simulink library "Eclipse"  (R2014b)
settings: Solver=ode45  StartTime=0.0  StopTime=10.0  RelTol=1e-3
undefined symbols (not defined in the file): ConfParam
settings Model: Creator=Hp  LastModifiedBy=Hp

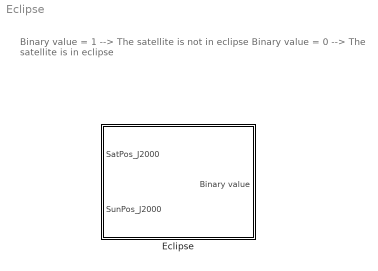
== system Eclipse ==
  note: Binary value = 1 --> The satellite is not in eclipse
      |
      | Binary value = 0 --> The satellite is in eclipse
  Eclipse : Subsystem

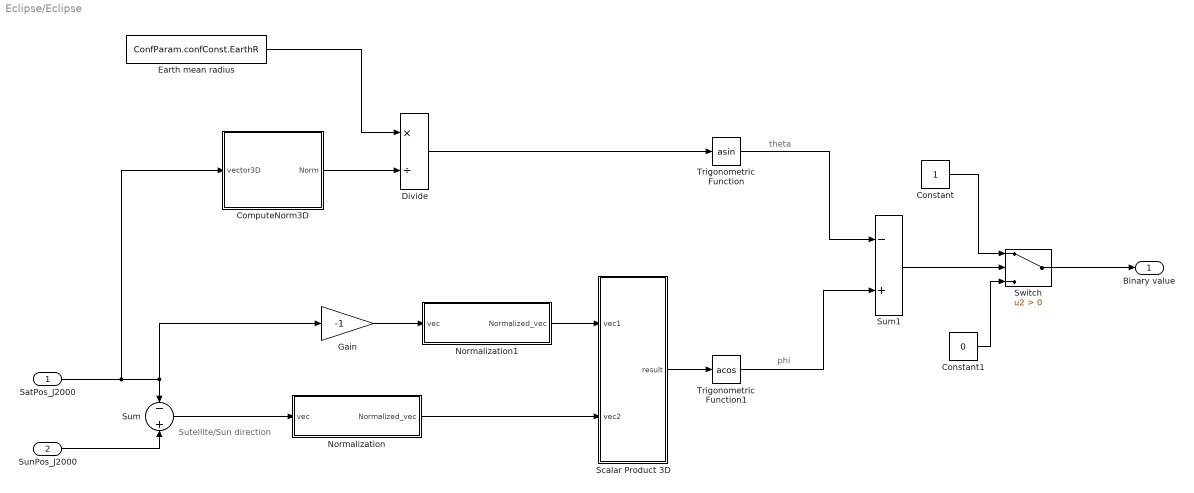
== system Eclipse/Eclipse ==
  note: phi
  note: theta
  note: Sutellite/Sun direction
  SatPos_J2000 : Inport
  SunPos_J2000 : Inport  Port=2
  ComputeNorm3D : Subsystem
  Constant : Constant
  Constant1 : Constant  Value=0
  Divide : Product  Inputs=*/
  Earth mean radius : Constant  Value=ConfParam.confConst.EarthR
  Gain : Gain  Gain=-1
  Normalization : Subsystem
  Normalization1 : Subsystem
  Scalar Product 3D : Subsystem
  Sum : Sum  Inputs=-|+
  Sum1 : Sum  Inputs=-+
  Switch : Switch  Criteria=u2 > Threshold
  Trigonometric Function : Trigonometry  Operator=asin
  Trigonometric Function1 : Trigonometry  Operator=acos
  Binary value : Outport
  wires:
  SatPos_J2000/1 -> ComputeNorm3D/1(vector3D), Sum/1, Gain/1
  SunPos_J2000/1 -> Sum/2
  Earth mean radius/1 -> Divide/1
  ComputeNorm3D/1(Norm) -> Divide/2
  Divide/1 -> Trigonometric Function/1
  Scalar Product 3D/1(result) -> Trigonometric Function1/1
  Sum/1 -> Normalization/1(vec)
  Normalization1/1(Normalized_vec) -> Scalar Product 3D/1(vec1)
  Normalization/1(Normalized_vec) -> Scalar Product 3D/2(vec2)
  Gain/1 -> Normalization1/1(vec)
  Switch/1 -> Binary value/1
  Trigonometric Function1/1 -> Sum1/2
  Constant/1 -> Switch/1
  Constant1/1 -> Switch/3
  Sum1/1 -> Switch/2
  Trigonometric Function/1 -> Sum1/1

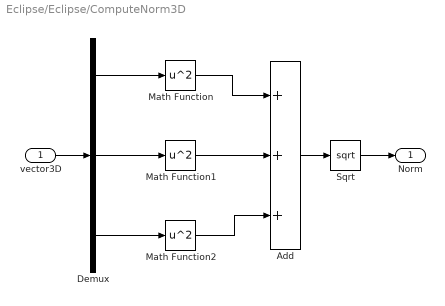
== system Eclipse/Eclipse/ComputeNorm3D ==
  vector3D : Inport
  Add : Sum  Inputs=+++
  Demux : Demux  Outputs=3
  Math Function : Math  Operator=square  SaturateOnIntegerOverflow=on
  Math Function1 : Math  Operator=square  SaturateOnIntegerOverflow=on
  Math Function2 : Math  Operator=square  SaturateOnIntegerOverflow=on
  Sqrt : Sqrt  SaturateOnIntegerOverflow=on
  Norm : Outport
  wires:
  vector3D/1 -> Demux/1
  Sqrt/1 -> Norm/1
  Add/1 -> Sqrt/1
  Math Function1/1 -> Add/2
  Math Function2/1 -> Add/3
  Demux/1 -> Math Function/1
  Math Function/1 -> Add/1
  Demux/3 -> Math Function2/1
  Demux/2 -> Math Function1/1

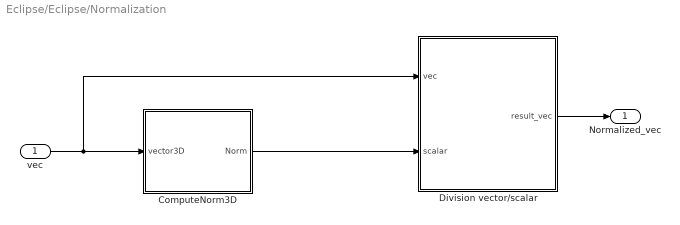
== system Eclipse/Eclipse/Normalization ==
  vec : Inport
  ComputeNorm3D : Subsystem
  Division vector/scalar : Subsystem
  Normalized_vec : Outport
  wires:
  vec/1 -> Division vector/scalar/1(vec), ComputeNorm3D/1(vector3D)
  Division vector/scalar/1(result_vec) -> Normalized_vec/1
  ComputeNorm3D/1(Norm) -> Division vector/scalar/2(scalar)

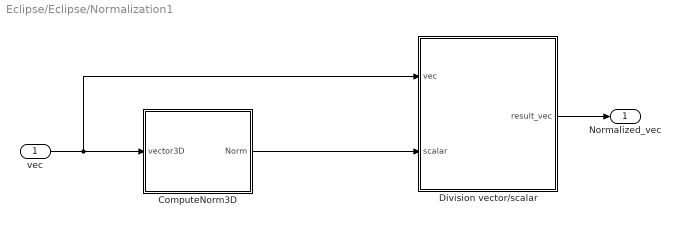
== system Eclipse/Eclipse/Normalization1 ==
  vec : Inport
  ComputeNorm3D : Subsystem
  Division vector/scalar : Subsystem
  Normalized_vec : Outport
  wires:
  vec/1 -> Division vector/scalar/1(vec), ComputeNorm3D/1(vector3D)
  Division vector/scalar/1(result_vec) -> Normalized_vec/1
  ComputeNorm3D/1(Norm) -> Division vector/scalar/2(scalar)

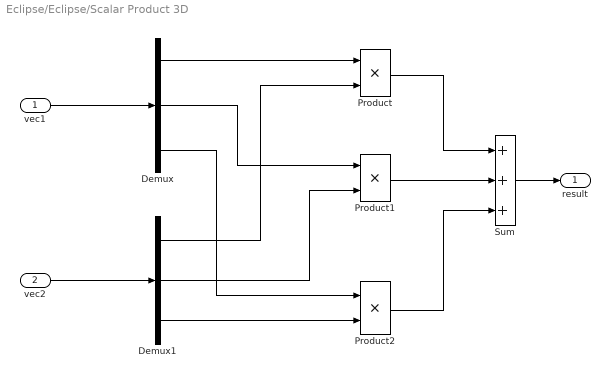
== system Eclipse/Eclipse/Scalar Product 3D ==
  vec1 : Inport
  vec2 : Inport  Port=2
  Demux : Demux  Outputs=3
  Demux1 : Demux  Outputs=3
  Product : Product
  Product1 : Product
  Product2 : Product
  Sum : Sum  Inputs=+++
  result : Outport
  wires:
  Product/1 -> Sum/1
  Demux/3 -> Product2/1
  Demux1/3 -> Product2/2
  Demux1/1 -> Product/2
  vec2/1 -> Demux1/1
  Product2/1 -> Sum/3
  Sum/1 -> result/1
  Demux/1 -> Product/1
  Demux/2 -> Product1/1
  Product1/1 -> Sum/2
  Demux1/2 -> Product1/2
  vec1/1 -> Demux/1

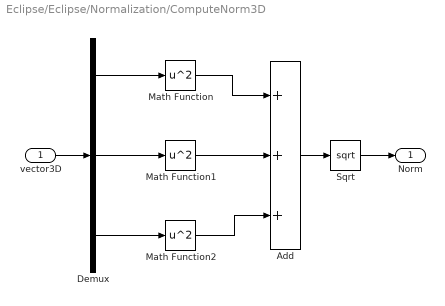
== system Eclipse/Eclipse/Normalization/ComputeNorm3D ==
  vector3D : Inport
  Add : Sum  Inputs=+++
  Demux : Demux  Outputs=3
  Math Function : Math  Operator=square  SaturateOnIntegerOverflow=on
  Math Function1 : Math  Operator=square  SaturateOnIntegerOverflow=on
  Math Function2 : Math  Operator=square  SaturateOnIntegerOverflow=on
  Sqrt : Sqrt  SaturateOnIntegerOverflow=on
  Norm : Outport
  wires:
  vector3D/1 -> Demux/1
  Sqrt/1 -> Norm/1
  Add/1 -> Sqrt/1
  Math Function1/1 -> Add/2
  Math Function2/1 -> Add/3
  Demux/1 -> Math Function/1
  Math Function/1 -> Add/1
  Demux/3 -> Math Function2/1
  Demux/2 -> Math Function1/1

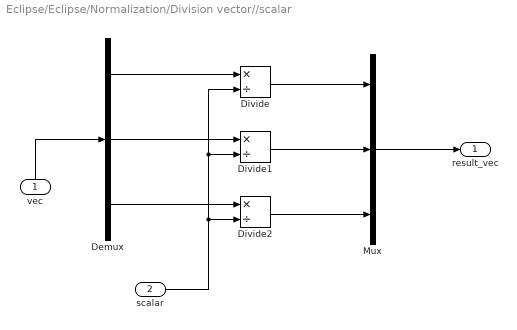
== system Eclipse/Eclipse/Normalization/Division vector//scalar ==
  vec : Inport
  scalar : Inport  Port=2
  Demux : Demux  Outputs=3
  Divide : Product  Inputs=*/
  Divide1 : Product  Inputs=*/
  Divide2 : Product  Inputs=*/
  Mux : Mux  Inputs=3
  result_vec : Outport
  wires:
  Divide/1 -> Mux/1
  Mux/1 -> result_vec/1
  scalar/1 -> Divide1/2, Divide/2, Divide2/2
  Demux/3 -> Divide2/1
  Divide2/1 -> Mux/3
  Divide1/1 -> Mux/2
  Demux/1 -> Divide/1
  Demux/2 -> Divide1/1
  vec/1 -> Demux/1

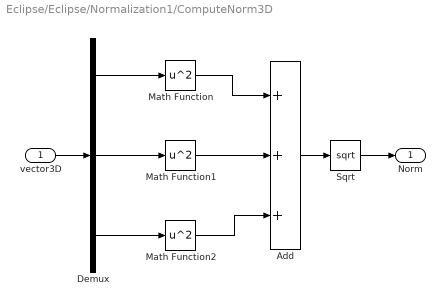
== system Eclipse/Eclipse/Normalization1/ComputeNorm3D ==
  vector3D : Inport
  Add : Sum  Inputs=+++
  Demux : Demux  Outputs=3
  Math Function : Math  Operator=square  SaturateOnIntegerOverflow=on
  Math Function1 : Math  Operator=square  SaturateOnIntegerOverflow=on
  Math Function2 : Math  Operator=square  SaturateOnIntegerOverflow=on
  Sqrt : Sqrt  SaturateOnIntegerOverflow=on
  Norm : Outport
  wires:
  vector3D/1 -> Demux/1
  Sqrt/1 -> Norm/1
  Add/1 -> Sqrt/1
  Math Function1/1 -> Add/2
  Math Function2/1 -> Add/3
  Demux/1 -> Math Function/1
  Math Function/1 -> Add/1
  Demux/3 -> Math Function2/1
  Demux/2 -> Math Function1/1

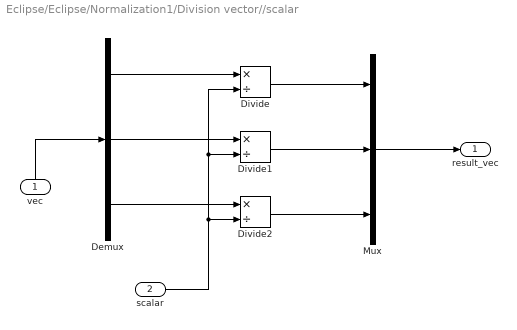
== system Eclipse/Eclipse/Normalization1/Division vector//scalar ==
  vec : Inport
  scalar : Inport  Port=2
  Demux : Demux  Outputs=3
  Divide : Product  Inputs=*/
  Divide1 : Product  Inputs=*/
  Divide2 : Product  Inputs=*/
  Mux : Mux  Inputs=3
  result_vec : Outport
  wires:
  Divide/1 -> Mux/1
  Mux/1 -> result_vec/1
  scalar/1 -> Divide1/2, Divide/2, Divide2/2
  Demux/3 -> Divide2/1
  Divide2/1 -> Mux/3
  Divide1/1 -> Mux/2
  Demux/1 -> Divide/1
  Demux/2 -> Divide1/1
  vec/1 -> Demux/1
